simulink model "FactorialForLoop"  (R2021a)
settings: Solver=FixedStepDiscrete  StartTime=0.0  StopTime=10.0  RelTol=1e-3  EnableMultiTasking=on
settings Model: Creator=Mina  LastModifiedBy=Mina
settings DataIOCC: ReturnWorkspaceOutputs=off
settings OptimizationCC: DefaultParameterBehavior=Inlined  InlineInvariantSignals=on  EnableMemcpy=off  LifeSpan=1  EfficientTunableParamExpr=on
settings DebuggingCC: UnderspecifiedInitializationDetection=Classic  MergeDetectMultiDrivingBlocksExec=none  SFMachineParentedDataDiag=warning  ArithmeticOperatorsInVariantConditions=warning
settings ModelReferenceCC: PropagateSignalLabelsOutOfModel=off
settings SFSimCC: MATLABDynamicMemAlloc=off  CustomCodeUndefinedFunction=UseInterfaceOnly
settings RTWCC: SystemTargetFile=ert.tlc  GenCodeOnly=on  TemplateMakefile=ert_default_tmf  GenerateReport=on  IncludeHyperlinkInReport=on  LaunchReport=on  GenerateTraceInfo=on  GenerateTraceReport=on  GenerateTraceReportSl=on  GenerateTraceReportSf=on  GenerateTraceReportEml=on
settings CodeAppCC: ForceParamTrailComments=on  IgnoreCustomStorageClasses=off  OperatorAnnotations=on  SimulinkDataObjDesc=on  SFDataObjDesc=on  MATLABFcnDesc=on  InsertBlockDesc=on  StateflowObjectComments=on  MATLABSourceComments=on
settings ERTTargetCC: MultiwordLength=2048  GenerateSampleERTMain=on  InlinedParameterPlacement=NonHierarchical  ERTCustomFileTemplate=example_file_process.tlc

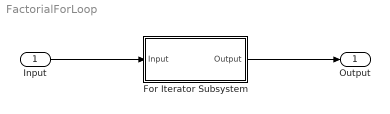
== system FactorialForLoop ==
  Input : Inport
  For Iterator Subsystem : Subsystem  TreatAsAtomicUnit=on
  Output : Outport
  wires:
  Input/1 -> For Iterator Subsystem/1(Input)
  For Iterator Subsystem/1(Output) -> Output/1

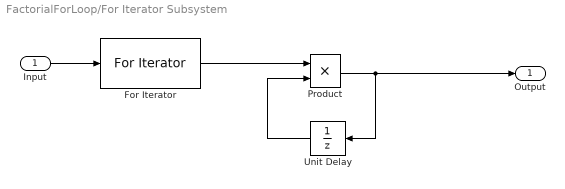
== system FactorialForLoop/For Iterator Subsystem ==
  Input : Inport  OutDataTypeStr=uint8
  For Iterator : ForIterator  IterationSource=external  IterationVariableDataType=uint8
  Product : Product  OutDataTypeStr=uint16  RndMeth=Nearest
  Unit Delay : UnitDelay  InitialCondition=1  SampleTime=-1  HasFrameUpgradeWarning=on
  Output : Outport  OutDataTypeStr=uint16
  wires:
  Product/1 -> Unit Delay/1, Output/1
  Unit Delay/1 -> Product/2
  For Iterator/1 -> Product/1
  Input/1 -> For Iterator/1
